simulink model "MATLAB_Func_u2"  (R2020b)
settings: Solver=VariableStepAuto  StartTime=0.0  StopTime=10.0  RelTol=1e-3
settings Model: Creator=ShiningDanyang  LastModifiedBy=ShiningDanyang

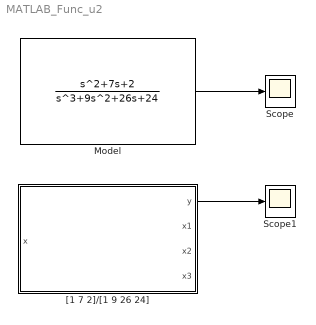
== system MATLAB_Func_u2 ==
  Model : TransferFcn  Numerator=[1 7 2]  Denominator=[1 9 26 24]
  Scope : Scope
  Scope1 : Scope
  "[1 7 2]/[1 9 26 24]" : Subsystem
  wires:
  "[1 7 2]/[1 9 26 24]"/1(y) -> Scope1/1
  Model/1 -> Scope/1

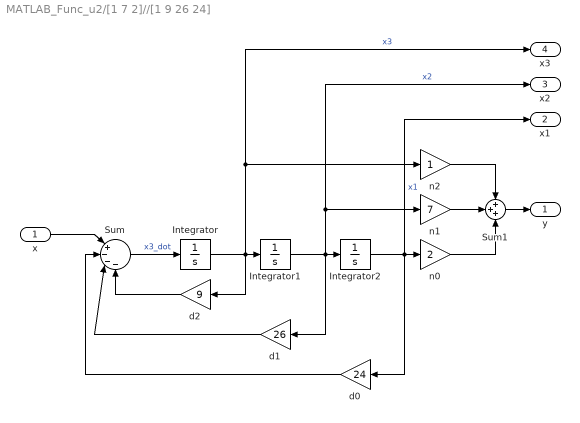
== system MATLAB_Func_u2/[1 7 2]//[1 9 26 24] ==
  x : Inport
  Integrator : Integrator
  Integrator1 : Integrator
  Integrator2 : Integrator
  Sum : Sum  Inputs=|+---
  Sum1 : Sum  Inputs=+++
  d0 : Gain  Gain=24
  d1 : Gain  Gain=26
  d2 : Gain  Gain=9
  n0 : Gain  Gain=2
  n1 : Gain  Gain=7
  n2 : Gain
  y : Outport
  x1 : Outport  Port=2
  x2 : Outport  Port=3
  x3 : Outport  Port=4
  wires:
  d0/1 -> Sum/2
  Sum/1 -> Integrator/1  "x3_dot"
  Integrator1/1 -> x2/1, n1/1, d1/1, Integrator2/1  "x2"
  d2/1 -> Sum/4
  Integrator2/1 -> x1/1, d0/1, n0/1  "x1"
  Integrator/1 -> x3/1, n2/1, d2/1, Integrator1/1  "x3"
  d1/1 -> Sum/3
  x/1 -> Sum/1
  n0/1 -> Sum1/3
  n1/1 -> Sum1/2
  Sum1/1 -> y/1
  n2/1 -> Sum1/1
